simulink model "NewKitchen_REB_workstation"  (R2020b)
settings: Solver=FixedStepAuto  StartTime=sim_start  StopTime=sim_end  FixedStep=sim_interval  RelTol=1e-3
undefined symbols (not defined in the file): AmbientTem, Power1, Power2, Power3, Velocity1, Velocity2
libraries: dspswit3 x6
(part 3 of 3)

== matlab function NewKitchen_REB_workstation/Signals/Power1/MATLAB Function ==
  data: num input; P1 output
function P1 = motion(num)
    
    N = ceil(num/30); 
    
    if N == 1
        P1 = 1000; % 5 + 3
    elseif N == 2
        P1 = 500; % 3 + 3
    elseif N == 3
        P1 = 0; % 2 + 3
    elseif N == 4
        P1 = 500; % 7 + 3
    elseif N == 5
        P1 = 1000; % 6 + 3
    elseif N == 6
        P1 = 500; % 4 + 3
    else
        P1 = 1000;
    end
    
end

== matlab function NewKitchen_REB_workstation/Signals/Power2/MATLAB Function ==
  data: num input; P2 output
function P2 = motion(num)
    
    N = ceil(num/30); 
    
    if N == 1
        P2 = 500; % 5 + 3
    elseif N == 2
        P2 = 1000; % 3 + 3
    elseif N == 3
        P2 = 200; % 2 + 3
    elseif N == 4
        P2 = 800; % 7 + 3
    elseif N == 5
        P2 = 600; % 6 + 3
    elseif N == 6
        P2 = 1000; % 4 + 3
    else
        P2 = 1000;
    end
    
end

== matlab function NewKitchen_REB_workstation/Signals/Power3/MATLAB Function ==
  data: num input; P3 output
function P3 = motion(num)
    
    N = ceil(num/30); 
    
    if N == 1
        P3 = 200; % 5 + 3
    elseif N == 2
        P3 = 600; % 3 + 3
    elseif N == 3
        P3 = 1000; % 2 + 3
    elseif N == 4
        P3 = 500; % 7 + 3
    elseif N == 5
        P3 = 0; % 6 + 3
    elseif N == 6
        P3 = 600; % 4 + 3
    else
        P3 = 1000;
    end
    
end

== matlab function NewKitchen_REB_workstation/Signals/V1/MATLAB Function ==
  data: num input; V1 output
function V1 = motion(num)
    
    N = ceil(num/30); 
    
    if N == 1
        V1 = 2; % 5 + 3
    elseif N == 2
        V1 = 0; % 3 + 3
    elseif N == 3
        V1 = 2; % 2 + 3
    elseif N == 4
        V1 = 0; % 7 + 3
    elseif N == 5
        V1 = 2; % 6 + 3
    elseif N == 6
        V1 = 0; % 4 + 3
    else
        V1 = 2;
    end
    
end

== matlab function NewKitchen_REB_workstation/Signals/V2/MATLAB Function ==
  data: num input; V2 output
function V2 = motion(num)
    
    N = ceil(num/30); 
    
    if N == 1
        V2 = 1; % 5 + 3
    elseif N == 2
        V2 = 0; % 3 + 3
    elseif N == 3
        V2 = 1; % 2 + 3
    elseif N == 4
        V2 = 0; % 7 + 3
    elseif N == 5
        V2 = 1; % 6 + 3
    elseif N == 6
        V2 = 0; % 4 + 3
    else
        V2 = 1;
    end
    
end

== matlab function NewKitchen_REB_workstation/Signals/AmbientTem/MATLAB Function ==
  data: num input; Tout output
function Tout = motion(num)

    Tout = randi([10,18]);

%    N = ceil(num/30); 
%     
%     if N == 1
%         Tout = 18; % 5 + 3
%     elseif N == 2
%         Tout = 16; % 3 + 3
%     elseif N == 3
%         Tout = 14; % 2 + 3
%     elseif N == 4
%         Tout = 12; % 7 + 3
%     elseif N == 5
%         Tout = 14; % 6 + 3
%     elseif N == 6
%         Tout = 16; % 4 + 3
%     else
%         Tout = 18;
%     end
    
end
